simulink model "Controlador_PID_final"  (Simulink 8.0)
settings: Solver=ode45  StartTime=0.0  StopTime=200  RelTol=1e-3
values from neighbouring files (symbols this model uses):
  a_lh_max = 1    [Parametros.m]
  a_lh_min = -1    [Parametros.m]
  a_xt_max = 1    [Parametros.m]
  a_xt_min = -1    [Parametros.m]
  bh = (beqi*ni^2)/Rd^2    (= 28800)    [Parametros.m]    (also in Parametros_completo.m = 1e-05)
  bt = (beqt*nt^2)/Rw^2    (= 27000)    [Parametros.m]    (also in Parametros_completo.m = 1e-05)
  bw = 3e3    (= 3000)    [Parametros.m]    (also in Parametros_completo.m = 0)
  Fh0 = mL*g    (= 637429)    [Parametros.m]    (also in Parametros_completo.m)
  g = 9.8066    [Parametros.m]    (also in Parametros_completo.m)
  kdx = (2*E*wn-p1x)*Mt-bt    (= 91016)    [Parametros.m]    (also in Parametros_completo.m = 2999999.99999)
  kdy = (2*E*wn-p1y)*Mh-bh + 9e4    (= 66001.4222222)    [Parametros.m]    (also in Parametros_completo.m = 20091.417269)
  kix = (-p1x*wn^2*Mt)    (= 59008)    [Parametros.m]    (also in Parametros_completo.m = 337500000)
  kiy = (-p1y*wn^2*Mh)/1e5    (= 60017.7777778)    [Parametros.m]    (also in Parametros_completo.m = 282535.555556)
  kpx = (wn^2-2*E*wn*p1x)*Mt    (= 118016)    [Parametros.m]    (also in Parametros_completo.m = 45000000)
  kpy = (wn^2-2*E*wn*p1y)*Mh    (= 240071.111111)    [Parametros.m]    (also in Parametros_completo.m = 216610.592593)
  Kw = 180e3    (= 180000)    [Parametros.m]    (also in Parametros_completo.m = 15935.725)
  lh_g = yt0 + yl_min -  (hContainer*numContainer(numColumna)) -mL*g/Kw    [Parametros.m]
  lh_h = yt0-yl0-mL*g/Kw    (= 35.4587277778)    [Parametros.m]
  lh_min = yt0 - yl_max-mL*g/Kw    (= 1.45872777778)    [Parametros.m]
  marg_lh = 5    [Parametros.m]
  marg_lh_g = 10    [Parametros.m]
  marg_xt = 5    [Parametros.m]
  marg_xt_g = 10    [Parametros.m]
  Mh = (Jd + Jm*ni^2)/Rd^2    (= 48014.2222222)    [Parametros.m]    (also in Parametros_completo.m = 125.571358025)
  mL = m0+ml    (= 65000)    [Parametros.m]    (also in Parametros_completo.m)
  Mt = (Mc + (Jw + Jmotort*nt^2)/Rw^2)    (= 59008)    [Parametros.m]    (also in Parametros_completo.m = 100000)
  ni = 30    [Parametros.m]    (also in Parametros_completo.m)
  nt = 15    [Parametros.m]    (also in Parametros_completo.m)
  Rd = 0.75    [Parametros.m]
  Rw = 0.5    [Parametros.m]
  Ts = (1/wn)/10    (= 0.002)    [Parametros.m]    (also in Parametros_completo.m = 0.00666666666667)
  v_lh_max = 1.5    [Parametros.m]
  v_lh_min = -1.5    [Parametros.m]
  v_xt_max = 1.5    [Parametros.m]
  v_xt_min = -1.5    [Parametros.m]
  xt_g = (numColumna + 0.5) * wContainer    (= 27.5)    [Parametros.m]
  xt_h = -15.0    (= -15)    [Parametros.m]
  yl0 = hContainer + 1    (= 6)    [Parametros.m]    (also in Parametros_completo.m = 0)
  yt0 = 45    [Parametros.m]    (also in Parametros_completo.m = 40)
libraries: simulink x1
settings Model: Creator=maximiliano  LastModifiedBy=alvaro
settings DataIOCC: SignalLoggingSaveFormat=ModelDataLogs
settings DebuggingCC: FcnCallInpInsideContextMsg=UseLocalSettings
settings GRTTargetCC: CombineOutputUpdateFcns=off  GRTInterface=on

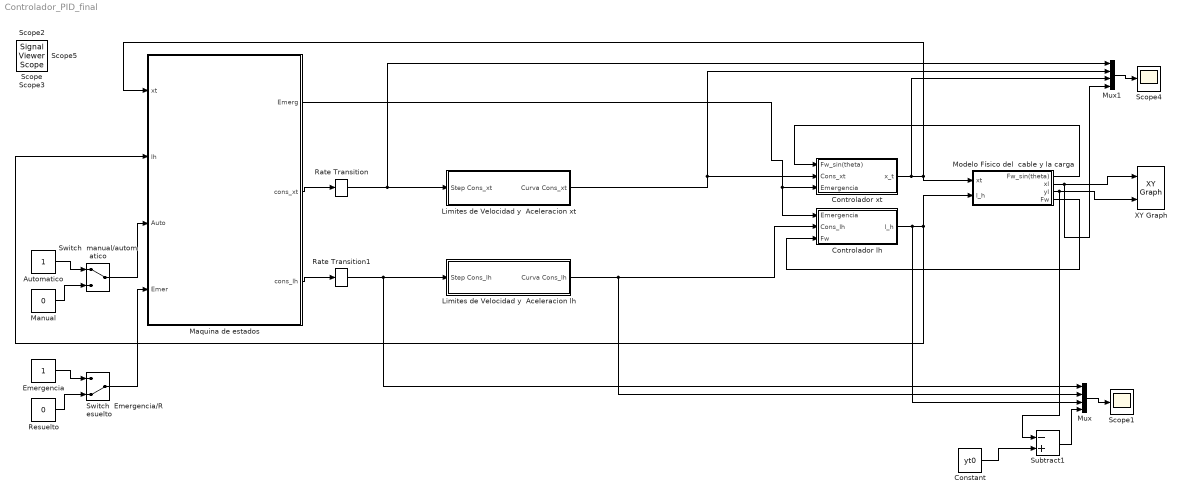
== system Controlador_PID_final ==
  Automatico : Constant
  Constant : Constant  Value=yt0
  Controlador lh : Subsystem
  Controlador xt : Subsystem
  Emergencia : Constant
  Limites de Velocidad y  Aceleracion lh : Subsystem
  Limites de Velocidad y  Aceleracion xt : Subsystem
  Manual : Constant  Value=0
  Maquina de estados : Stateflow chart  RequirementInfo={'other' '' '' 'true' '' '' } %GIDa_ef387a8e_3621_4cf2_ab41_fec22cdb0742  TreatAsAtomicUnit=on
  Modelo Físico del  cable y la carga : Subsystem
  Mux : Mux
  Mux1 : Mux
  Rate Transition : RateTransition  OutPortSampleTime=Ts
  Rate Transition1 : RateTransition  OutPortSampleTime=Ts
  Resuelto : Constant  Value=0
  Scope1 : Scope
      settings: TimeRange=200  YMin=0  YMax=65
  Scope4 : Scope
      settings: TimeRange=200  YMin=-20  YMax=30
  Subtract1 : Sum  Inputs=-+
  Switch  Emergencia/Resuelto : ManualSwitch  CurrentSetting=0
  Switch  manual/automatico : ManualSwitch
  XY Graph : simulink/Sinks/XY Graph  xmin=-40  xmax=60  ymin=-30  ymax=50  st=-1
  Scope : SignalViewerScope  IOType=viewer  RefreshTime=0.035000
  Scope2 : SignalViewerScope  IOType=viewer  ZoomMode=yonly  RefreshTime=0.035000
      settings: YMin=5e-11  YMax=4.75e-10  SaveName=ScopeData2
  Scope3 : SignalViewerScope  IOType=viewer  RefreshTime=0.035000
      settings: YMin=-0.00012  YMax=0.0001  SaveName=ScopeData3
  Scope5 : SignalViewerScope  IOType=viewer  RefreshTime=0.035000
  wires:
  Controlador xt/1(x_t) -> Mux1/3, Maquina de estados/1(xt), Modelo Físico del  cable y la carga/1(xt)
  Controlador lh/1(l_h) -> Mux/3, Maquina de estados/2(lh), Modelo Físico del  cable y la carga/2(l_h)
  Modelo Físico del  cable y la carga/4(Fw) -> Controlador lh/3(Fw)
  Modelo Físico del  cable y la carga/1(Fw_sin(theta)) -> Controlador xt/1(Fw_sin(theta))
  Maquina de estados/1(Emerg) -> Controlador lh/1(Emergencia), Controlador xt/3(Emergencia)
  Automatico/1 -> Switch  manual/automatico/1
  Manual/1 -> Switch  manual/automatico/2
  Switch  manual/automatico/1 -> Maquina de estados/3(Auto)
  Modelo Físico del  cable y la carga/2(xl) -> Mux1/4, XY Graph/1
  Modelo Físico del  cable y la carga/3(yl) -> Subtract1/1, XY Graph/2
  Maquina de estados/3(cons_lh) -> Rate Transition1/1
  Limites de Velocidad y  Aceleracion lh/1(Curva Cons_lh) -> Mux/2, Controlador lh/2(Cons_lh)
  Maquina de estados/2(cons_xt) -> Rate Transition/1
  Limites de Velocidad y  Aceleracion xt/1(Curva Cons_xt) -> Mux1/2, Controlador xt/2(Cons_xt)
  Rate Transition/1 -> Limites de Velocidad y  Aceleracion xt/1(Step Cons_xt), Mux1/1
  Rate Transition1/1 -> Limites de Velocidad y  Aceleracion lh/1(Step Cons_lh), Mux/1
  Mux/1 -> Scope1/1
  Constant/1 -> Subtract1/2
  Subtract1/1 -> Mux/4
  Mux1/1 -> Scope4/1
  Emergencia/1 -> Switch  Emergencia/Resuelto/1
  Resuelto/1 -> Switch  Emergencia/Resuelto/2
  Switch  Emergencia/Resuelto/1 -> Maquina de estados/4(Emer)

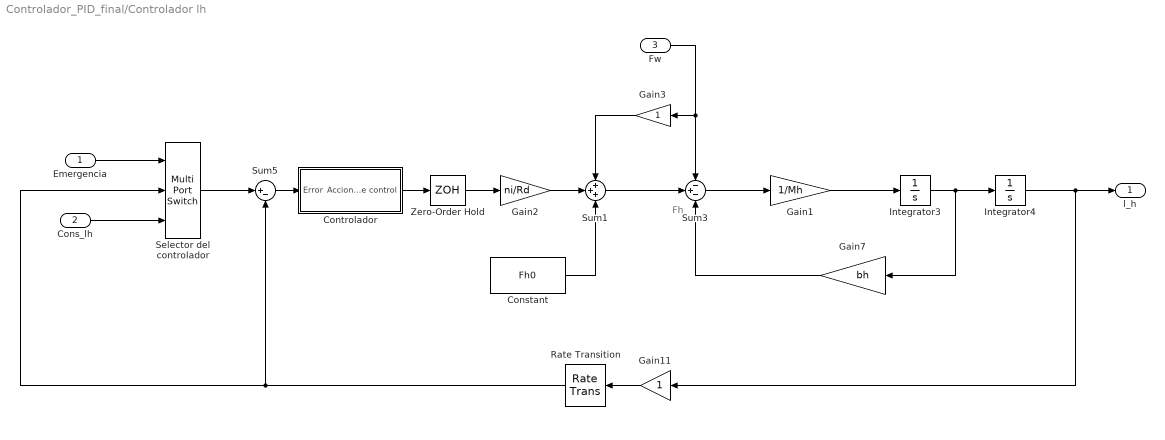
== system Controlador_PID_final/Controlador lh ==
  note: Fh
  Emergencia : Inport
  Cons_lh : Inport  Port=2
  Fw : Inport  Port=3
  Constant : Constant  Value=Fh0
  Controlador : Subsystem
  Gain1 : Gain  Gain=1/Mh
  Gain11 : Gain
  Gain2 : Gain  Gain=ni/Rd
  Gain3 : Gain
  Gain7 : Gain  Gain=bh
  Integrator3 : Integrator
  Integrator4 : Integrator  InitialCondition=lh_h
  Rate Transition : RateTransition  OutPortSampleTime=Ts
  Selector del controlador : MultiPortSwitch  Inputs=2
  Sum1 : Sum  Inputs=+++
  Sum3 : Sum  Inputs=-+-
  Sum5 : Sum  Inputs=|+-
  Zero-Order Hold : ZeroOrderHold  SampleTime=Ts
  l_h : Outport
  wires:
  Gain1/1 -> Integrator3/1
  Integrator3/1 -> Integrator4/1, Gain7/1
  Integrator4/1 -> l_h/1, Gain11/1
  Gain7/1 -> Sum3/3
  Sum3/1 -> Gain1/1
  Gain11/1 -> Rate Transition/1
  Rate Transition/1 -> Sum5/2, Selector del controlador/2
  Controlador/1(Accion de control) -> Zero-Order Hold/1
  Zero-Order Hold/1 -> Gain2/1
  Fw/1 -> Sum3/1, Gain3/1
  Gain3/1 -> Sum1/1
  Constant/1 -> Sum1/3
  Selector del controlador/1 -> Sum5/1
  Emergencia/1 -> Selector del controlador/1
  Cons_lh/1 -> Selector del controlador/3
  Sum5/1 -> Controlador/1(Error)
  Gain2/1 -> Sum1/2
  Sum1/1 -> Sum3/2

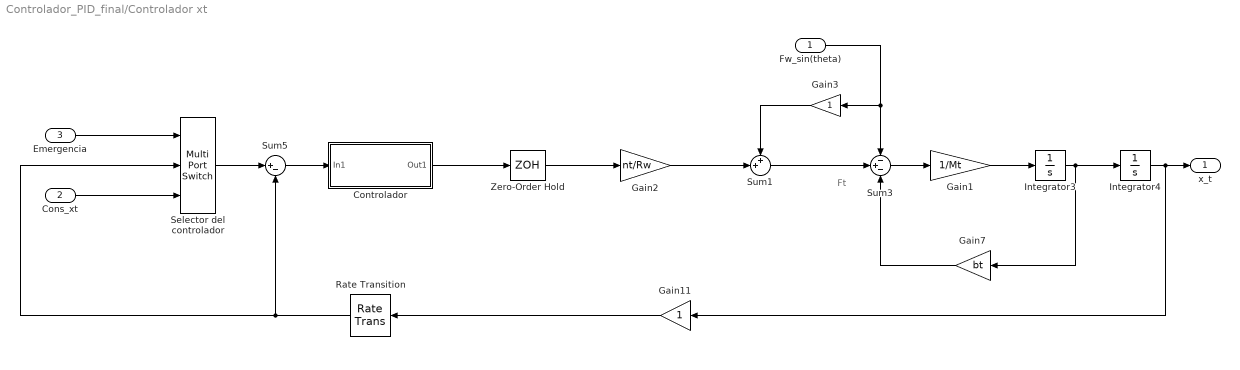
== system Controlador_PID_final/Controlador xt ==
  note: Ft
  Fw_sin(theta) : Inport
  Cons_xt : Inport  Port=2
  Emergencia : Inport  Port=3
  Controlador : Subsystem
  Gain1 : Gain  Gain=1/Mt
  Gain11 : Gain
  Gain2 : Gain  Gain=nt/Rw
  Gain3 : Gain
  Gain7 : Gain  Gain=bt
  Integrator3 : Integrator
  Integrator4 : Integrator  InitialCondition=xt_h
  Rate Transition : RateTransition  OutPortSampleTime=Ts
  Selector del controlador : MultiPortSwitch  Inputs=2
  Sum1 : Sum  Inputs=++|  SampleTime=Ts
  Sum3 : Sum  Inputs=-+-
  Sum5 : Sum  Inputs=|+-
  Zero-Order Hold : ZeroOrderHold  SampleTime=Ts
  x_t : Outport
  wires:
  Gain1/1 -> Integrator3/1
  Integrator3/1 -> Integrator4/1, Gain7/1
  Integrator4/1 -> Gain11/1, x_t/1
  Gain7/1 -> Sum3/3
  Sum3/1 -> Gain1/1
  Gain11/1 -> Rate Transition/1
  Rate Transition/1 -> Sum5/2, Selector del controlador/2
  Zero-Order Hold/1 -> Gain2/1
  Fw_sin(theta)/1 -> Sum3/1, Gain3/1
  Gain3/1 -> Sum1/1
  Selector del controlador/1 -> Sum5/1
  Emergencia/1 -> Selector del controlador/1
  Cons_xt/1 -> Selector del controlador/3
  Sum5/1 -> Controlador/1(In1)
  Controlador/1(Out1) -> Zero-Order Hold/1
  Gain2/1 -> Sum1/2
  Sum1/1 -> Sum3/2

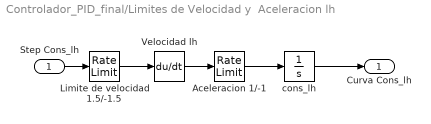
== system Controlador_PID_final/Limites de Velocidad y  Aceleracion lh ==
  Step Cons_lh : Inport
  Aceleracion 1/-1 : RateLimiter  RisingSlewLimit=a_lh_max  FallingSlewLimit=a_lh_min  SampleTimeMode=inherited
  Limite de velocidad 1.5/-1.5 : RateLimiter  RisingSlewLimit=v_lh_max  FallingSlewLimit=v_lh_min  SampleTimeMode=inherited  InitialCondition=lh_h
  Velocidad lh : Derivative  CoefficientInTFapproximation=1000
  cons_lh : Integrator  InitialCondition=lh_h
  Curva Cons_lh : Outport
  wires:
  Velocidad lh/1 -> Aceleracion 1/-1/1
  Aceleracion 1/-1/1 -> cons_lh/1
  Limite de velocidad 1.5/-1.5/1 -> Velocidad lh/1
  Step Cons_lh/1 -> Limite de velocidad 1.5/-1.5/1
  cons_lh/1 -> Curva Cons_lh/1

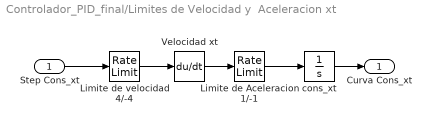
== system Controlador_PID_final/Limites de Velocidad y  Aceleracion xt ==
  Step Cons_xt : Inport
  "Limite de Aceleracion 1/-1 " : RateLimiter  RisingSlewLimit=a_xt_max  FallingSlewLimit=a_xt_min  SampleTimeMode=inherited
  "Limite de velocidad 4/-4 " : RateLimiter  RisingSlewLimit=v_xt_max  FallingSlewLimit=v_xt_min  SampleTimeMode=inherited  InitialCondition=xt_h
  Velocidad xt : Derivative
  cons_xt : Integrator  InitialCondition=xt_h
  Curva Cons_xt : Outport
  wires:
  cons_xt/1 -> Curva Cons_xt/1
  "Limite de velocidad 4/-4 "/1 -> Velocidad xt/1
  Velocidad xt/1 -> "Limite de Aceleracion 1/-1 "/1
  "Limite de Aceleracion 1/-1 "/1 -> cons_xt/1
  Step Cons_xt/1 -> "Limite de velocidad 4/-4 "/1

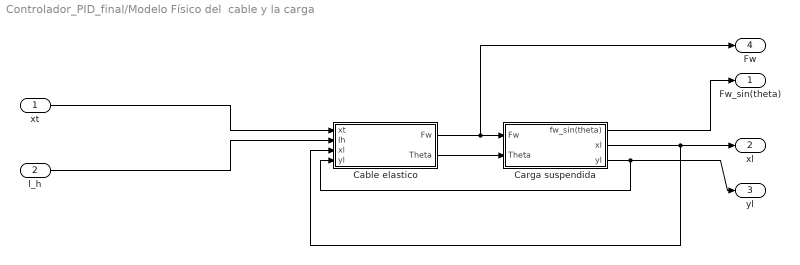
== system Controlador_PID_final/Modelo Físico del  cable y la carga ==
  xt : Inport
  l_h : Inport  Port=2
  Cable elastico : Subsystem
  Carga suspendida : Subsystem
  Fw_sin(theta) : Outport
  xl : Outport  Port=2
  yl : Outport  Port=3
  Fw : Outport  Port=4
  wires:
  Carga suspendida/3(yl) -> yl/1, Cable elastico/4(yl)
  Carga suspendida/2(xl) -> xl/1, Cable elastico/3(xl)
  xt/1 -> Cable elastico/1(xt)
  l_h/1 -> Cable elastico/2(Ih)
  Carga suspendida/1(fw_sin(theta)) -> Fw_sin(theta)/1
  Cable elastico/1(Fw) -> Carga suspendida/1(Fw), Fw/1
  Cable elastico/2(Theta) -> Carga suspendida/2(Theta)

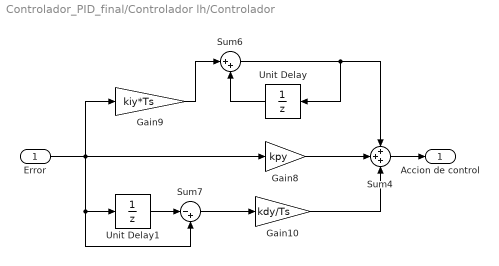
== system Controlador_PID_final/Controlador lh/Controlador ==
  Error : Inport
  Gain10 : Gain  Gain=kdy/Ts  SampleTime=Ts
  Gain8 : Gain  Gain=kpy  SampleTime=Ts
  Gain9 : Gain  Gain=kiy*Ts  SampleTime=Ts
  Sum4 : Sum  Inputs=+++
  Sum6 : Sum  Inputs=|++  SampleTime=Ts
  Sum7 : Sum  Inputs=|-+
  Unit Delay : UnitDelay  SampleTime=Ts
  Unit Delay1 : UnitDelay  SampleTime=Ts
  Accion de control : Outport
  wires:
  Error/1 -> Gain8/1, Gain9/1, Unit Delay1/1, Sum7/2
  Gain8/1 -> Sum4/2
  Gain10/1 -> Sum4/3
  Sum6/1 -> Sum4/1, Unit Delay/1
  Unit Delay1/1 -> Sum7/1
  Sum7/1 -> Gain10/1
  Unit Delay/1 -> Sum6/2
  Gain9/1 -> Sum6/1
  Sum4/1 -> Accion de control/1

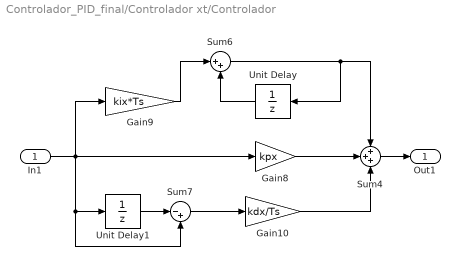
== system Controlador_PID_final/Controlador xt/Controlador ==
  In1 : Inport
  Gain10 : Gain  Gain=kdx/Ts  SampleTime=Ts
  Gain8 : Gain  Gain=kpx  SampleTime=Ts
  Gain9 : Gain  Gain=kix*Ts  SampleTime=Ts
  Sum4 : Sum  Inputs=+++
  Sum6 : Sum  Inputs=|++  SampleTime=Ts
  Sum7 : Sum  Inputs=|-+
  Unit Delay : UnitDelay  SampleTime=Ts
  Unit Delay1 : UnitDelay  SampleTime=Ts
  Out1 : Outport
  wires:
  In1/1 -> Gain8/1, Gain9/1, Unit Delay1/1, Sum7/2
  Gain8/1 -> Sum4/2
  Gain10/1 -> Sum4/3
  Sum6/1 -> Sum4/1, Unit Delay/1
  Unit Delay1/1 -> Sum7/1
  Sum7/1 -> Gain10/1
  Unit Delay/1 -> Sum6/2
  Gain9/1 -> Sum6/1
  Sum4/1 -> Out1/1

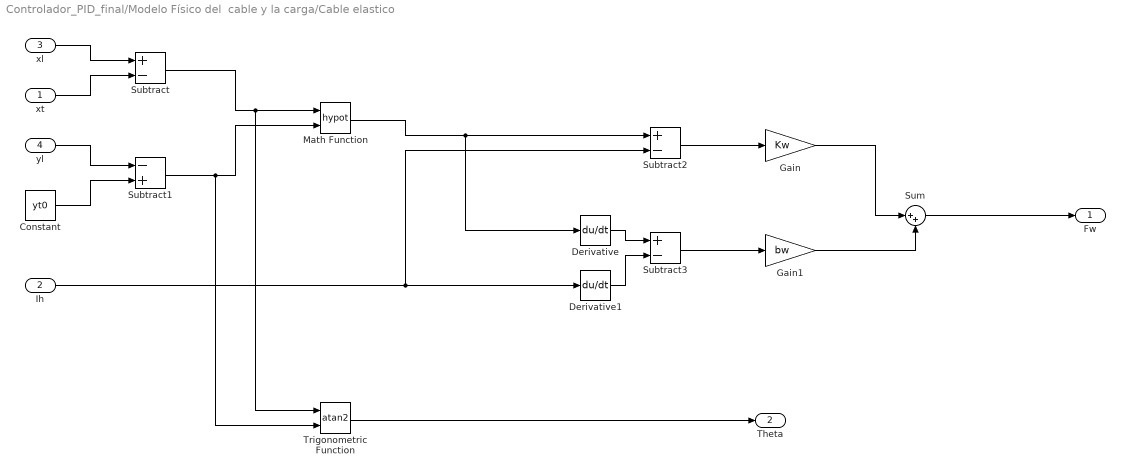
== system Controlador_PID_final/Modelo Físico del  cable y la carga/Cable elastico ==
  xt : Inport
  Ih : Inport  Port=2
  xl : Inport  Port=3
  yl : Inport  Port=4
  Constant : Constant  Value=yt0
  Derivative : Derivative
  Derivative1 : Derivative
  Gain : Gain  Gain=Kw
  Gain1 : Gain  Gain=bw
  Math Function : Math  Operator=hypot  SaturateOnIntegerOverflow=on
  Subtract : Sum  Inputs=+-
  Subtract1 : Sum  Inputs=-+
  Subtract2 : Sum  Inputs=+-
  Subtract3 : Sum  Inputs=+-
  Sum : Sum  Inputs=|++
  Trigonometric Function : Trigonometry  Operator=atan2
  Fw : Outport
  Theta : Outport  Port=2
  wires:
  xl/1 -> Subtract/1
  xt/1 -> Subtract/2
  Subtract/1 -> Math Function/1, Trigonometric Function/1
  yl/1 -> Subtract1/1
  Constant/1 -> Subtract1/2
  Subtract1/1 -> Math Function/2, Trigonometric Function/2
  Math Function/1 -> Subtract2/1, Derivative/1
  Ih/1 -> Subtract2/2, Derivative1/1
  Subtract2/1 -> Gain/1
  Gain/1 -> Sum/1
  Trigonometric Function/1 -> Theta/1
  Sum/1 -> Fw/1
  Subtract3/1 -> Gain1/1
  Derivative/1 -> Subtract3/1
  Derivative1/1 -> Subtract3/2
  Gain1/1 -> Sum/2

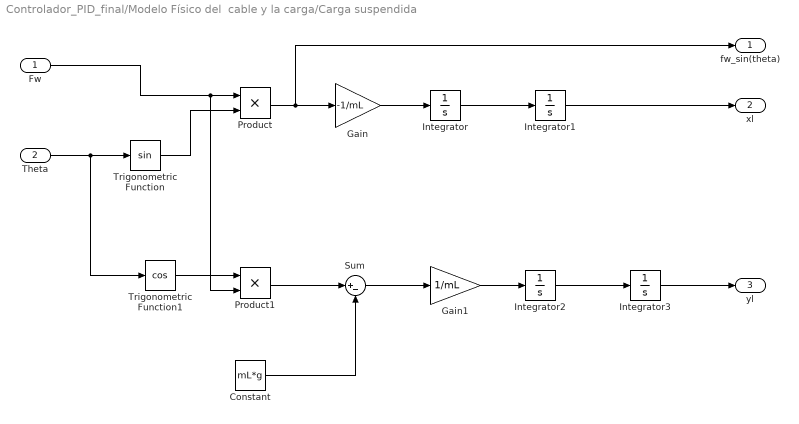
== system Controlador_PID_final/Modelo Físico del  cable y la carga/Carga suspendida ==
  Fw : Inport
  Theta : Inport  Port=2
  Constant : Constant  Value=mL*g
  Gain : Gain  Gain=-1/mL
  Gain1 : Gain  Gain=1/mL
  Integrator : Integrator
  Integrator1 : Integrator  InitialCondition=xt_h
  Integrator2 : Integrator
  Integrator3 : Integrator  InitialCondition=yl0
  Product : Product  RndMeth=Zero
  Product1 : Product  RndMeth=Zero
  Sum : Sum  Inputs=|+-
  Trigonometric Function : Trigonometry
  Trigonometric Function1 : Trigonometry  Operator=cos
  fw_sin(theta) : Outport
  xl : Outport  Port=2
  yl : Outport  Port=3
  wires:
  Theta/1 -> Trigonometric Function/1, Trigonometric Function1/1
  Fw/1 -> Product/1, Product1/2
  Trigonometric Function/1 -> Product/2
  Product/1 -> Gain/1, fw_sin(theta)/1
  Gain/1 -> Integrator/1
  Integrator/1 -> Integrator1/1
  Integrator1/1 -> xl/1
  Trigonometric Function1/1 -> Product1/1
  Product1/1 -> Sum/1
  Constant/1 -> Sum/2
  Sum/1 -> Gain1/1
  Gain1/1 -> Integrator2/1
  Integrator2/1 -> Integrator3/1
  Integrator3/1 -> yl/1

== stateflow chart Maquina de estados ==
  state Return
    cons_xt=xt_h;
    cons_lh=lh_min;
    Emerg = 2;
  state UpHome
    cons_xt=xt_h;
    cons_lh=lh_min;
    Emerg = 2;
  state DownHome
    cons_xt=xt_h;
    cons_lh=lh_h;
    Emerg = 2;
  state UpEnd
    cons_xt=xt_g;
    cons_lh=lh_min;
    Emerg = 2;
  state Go
    cons_xt=xt_g;
    cons_lh=lh_min;
    Emerg = 2;
  state Auto
    cons_xt=xt_h;
    cons_lh=lh_h;
    Emerg = 2;
  state DownEnd
    cons_xt=xt_g;
    cons_lh=lh_g;
    Emerg = 2;
  state End
    Emerg = 2;
  state AproachEnd
    cons_xt=xt_g;
    cons_lh=lh_g;
    Emerg = 2;
  state AproachHome
    cons_xt=xt_h;
    cons_lh=lh_h;
    Emerg = 2;
  state Emergency
    cons_xt=xt;
    cons_lh=lh;
    Emerg = 2;
  state Manual
    cons_xt=xt_h;
    cons_lh=lh_h;
    Emerg = 2;
  (default) -> Manual
  Emergency -> Manual : [Emer==0]
  End -> Manual [order 2] : [Auto==0]
  Manual -> Auto : [Auto==1]
  Auto -> AproachHome [order 2] : [marg_xt_g>=abs(xt-xt_h)]
  Auto -> AproachEnd [order 3] : [marg_xt_g>=abs(xt-xt_g)]
  Auto -> Emergency [order 1] : [marg_xt_g<=abs(xt-xt_h)|| marg_xt_g<=abs(xt-xt_g) ]
  AproachEnd -> Emergency [order 1] : [Emer==1]
  AproachHome -> Emergency [order 1] : [Emer==1]
  AproachEnd -> (junction 31) [order 2] : [after(50,tick)]
  AproachHome -> (junction 32) [order 2] : [after(5,sec)]
  (junction 31) -> Emergency [order 1] : [marg_xt_g<=abs(xt-xt_g)]
  (junction 32) -> Emergency [order 1] : [marg_xt_g<=abs(xt-xt_h)]
  (junction 31) -> UpEnd [order 2] : [marg_xt>=abs(xt-xt_g)]
  (junction 32) -> UpHome [order 2] : [marg_xt>=abs(xt-xt_h)]
  UpEnd -> Emergency [order 1] : [Emer==1]
  UpHome -> Emergency [order 1] : [Emer==1]
  UpHome -> (junction 33) [order 2] : [after(50,tick)]
  UpEnd -> (junction 34) [order 2] : [after(50,tick)]
  (junction 33) -> Emergency [order 1] : [abs(lh_h-lh_min)+1<=abs(lh-lh_min)]
  (junction 33) -> Go [order 2] : [marg_lh>=abs(lh-lh_min)]
  (junction 34) -> Emergency [order 1] : [abs(lh_g-lh_min)+1<=abs(lh-lh_min)]
  (junction 34) -> Return [order 2] : [marg_lh>=abs(lh-lh_min)]
  Go -> Emergency [order 1] : [Emer==1]
  Return -> Emergency [order 1] : [Emer==1]
  Go -> (junction 35) [order 2] : [after(50,tick)]
  Return -> (junction 36) [order 2] : [after(50,tick)]
  (junction 35) -> Emergency [order 1] : [abs(xt_h-xt_g)<=abs(xt-xt_g)]
  (junction 35) -> DownEnd [order 2] : [marg_xt>=abs(xt-xt_g)]
  (junction 36) -> Emergency [order 1] : [abs(xt_g-xt_h)<=abs(xt-xt_h)]
  (junction 36) -> DownHome [order 2] : [marg_xt>=abs(xt-xt_h)]
  (junction 37) -> Emergency [order 1] : [abs(lh_min-lh_g)+1<=abs(lh-lh_g)]
  DownEnd -> Emergency [order 1] : [Emer==1]
  End -> Emergency [order 1] : [Emer==1]
  DownHome -> Emergency [order 1] : [Emer==1]
  (junction 38) -> Emergency [order 1] : [abs(lh_min-lh_g)<=abs(lh-lh_h)]
  DownEnd -> (junction 37) [order 2] : [after(50,tick)]
  DownHome -> (junction 38) [order 2] : [after(50,tick)]
  (junction 37) -> End [order 2] : [marg_lh>=abs(lh-lh_g)]
  (junction 38) -> End [order 2] : [marg_lh>=abs(lh-lh_h)]
  data: Emerg output double; xt input double; lh input double; cons_xt output double; cons_lh output double; Auto input double; marg_lh parameter double; marg_lh_g parameter double; marg_xt parameter double; marg_xt_g parameter double; lh_g parameter double; lh_h parameter double; lh_min parameter double; xt_g parameter double; xt_h parameter double; Emer input double
